simulink model "AdaptiveModel"  (R2017b)
settings: Solver=VariableStepAuto  StartTime=0.0  StopTime=50  RelTol=1e-3
values from neighbouring files (symbols this model uses):
  beta = 40    [init.m]
  d = 1    [PP_rt.m]    (also in Poleplace.m; init.m)
  DT = 25    [init.m]
  Hr = [1 1]    [codegen.m]    (also in init.m)
  Hs = [1 -1]    [codegen.m]    (also in init.m)
  lambda = 0.95    [init.m]
  nA = length(A) - 1    [PP_rt_mauro.m]    (also in init.m)
  nB = length(B)    [PP_rt_mauro.m]    (also in init.m = length(B)-d-1)
  P = conv(P, Pf)    [PP_rt.m]    (also in PP_rt_mauro.m; codegen.m = [1 p1 p2]; init.m = [1 p1 p2])
  R1 = [33.5196767708 -58.8280554104 -1.87387669035 47.8358795149 0.399729759777 -15.7091995028 -25.6032753946 14.884365398 6.95997961448 3.86481013031 -6.742321562 4.41607857048 ... (17 elements, 1x17)]    [K1.mat]    (also in PP_rt.m = x(n_s1+2:end)'; Poleplace.m = x(n_s1+2:end)')
  R2 = [3.1342268844 -8.1399581872 5.33533955505 7.22995752468 -11.9866953907 -6.12499171015 23.0985636543 -12.1704635393 -4.51612658948 4.32936024322 -1.34202391707 6.4773700521 ... (17 elements, 1x17)]    [K2.mat]    (also in codegen.m = R_final)
  R3 = [3.98644760074 -10.644578896 12.4117237154 -5.12999859704 -6.58572397563 12.528754402 -9.78958840161 3.26868202994]    [K3.mat]    (also in K3_with_four_poles.mat = [1.61350975718 -4.21138815342 4.85167932198 -1.93039613093 -; init.m = [R3,0])
  S1 = [1 0.47525789568 -0.120791737843 -0.659025383432 -0.740602287059 -0.383041723471 0.0476399963873 0.338468948565 0.342443506099 0.181293316692 -0.0249270399759 -0.1387227703 ... (16 elements, 1x16)]    [K1.mat]    (also in PP_rt.m = x(1:n_s1+1)'; Poleplace.m = x(1:n_s1+1)')
  S2 = [1 -1.30861512012 -0.251094188933 0.310166607487 0.641482122367 -0.0760817308484 -0.446961768632 0.0650663960157 0.174068991686 -0.0320715572699 -0.0977287236514 -0.0172838591405 ... (16 elements, 1x16)]    [K2.mat]    (also in codegen.m = S_final)
  S3 = [1 -1.72076165185 1.25933960301 -0.482682162577 0.0902319524628 -0.117297255986 -0.0288304850576]    [K3.mat]    (also in K3_with_four_poles.mat = [1 -2.32113674008 2.28108582065 -1.19868534637 0.34993218961; init.m = [S3,0])
  Ts = 0.04    [codegen.m]    (also in init.m; p1p2.m)
libraries: cstblocks x3, simulink x1
settings Model: Creator=akarimi  LastModifiedBy=stenelling
settings CodeAppCC: StateflowObjectComments=on

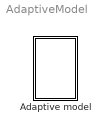
== system AdaptiveModel ==
  Adaptive model : Subsystem

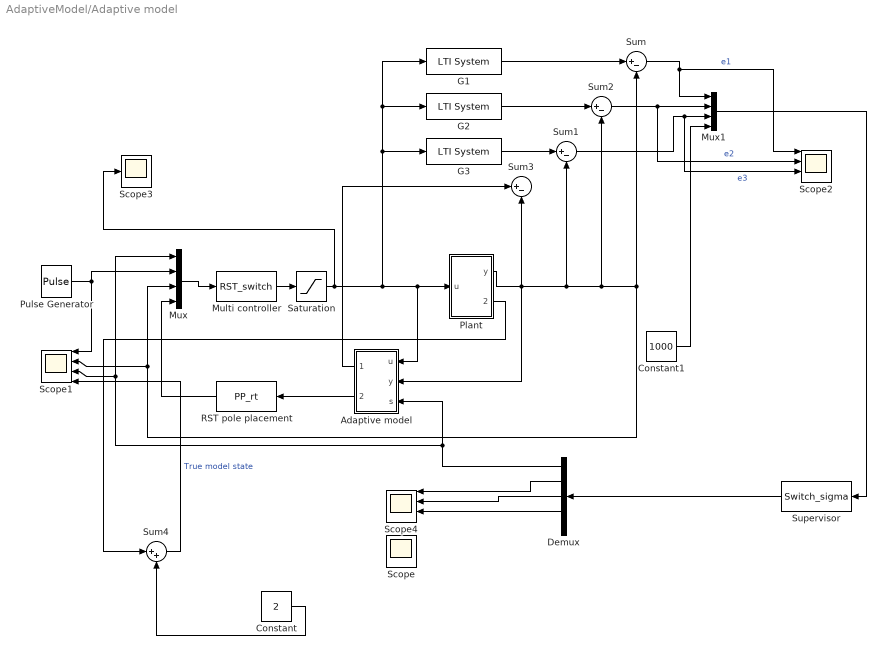
== system AdaptiveModel/Adaptive model ==
  Adaptive model : Subsystem
  Constant : Constant  Value=2
  Constant1 : Constant  Value=1000
  Demux : Demux  Outputs=5
  G1 : cstblocks/LTI System  sys=G1  IC=[]
  G2 : cstblocks/LTI System  sys=G2  IC=[]
  G3 : cstblocks/LTI System  sys=G3  IC=[]
  Multi controller : S-Function  FunctionName=RST_switch  Parameters=R1,S1,R2,S2,R3,S3,Ts  SFunctionDeploymentMode=off  EnableBusSupport=off
  Mux : Mux
  Mux1 : Mux
  Plant : Subsystem
  Pulse Generator : DiscretePulseGenerator  PulseType=Time based  Period=10  PulseWidth=50  PhaseDelay=5
  RST pole placement : S-Function  FunctionName=PP_rt  Parameters=nA,nB,d,P,Hs,Hr,Ts  SFunctionModules='Poleplace'  SFunctionDeploymentMode=off  EnableBusSupport=off
  Saturation : Saturate  UpperLimit=2  LowerLimit=-2
  Scope : Scope
  Scope1 : Scope  NumInputPorts=4
  Scope2 : Scope  NumInputPorts=4
  Scope3 : Scope
  Scope4 : Scope  NumInputPorts=4
  Sum{,1..3} (4 alike) : Sum  Inputs=|+-
  Sum4 : Sum  Inputs=|++
  Supervisor : S-Function  FunctionName=Switch_sigma  Parameters=beta,lambda,DT  SFunctionDeploymentMode=off  EnableBusSupport=off
  wires:
  Mux/1 -> Multi controller/1
  RST pole placement/1 -> Mux/4
  Pulse Generator/1 -> Scope1/1, Mux/2
  Plant/1(y) -> Adaptive model/2(y), Sum3/2, Scope1/2, Mux/3, Sum/2, Sum2/2, Sum1/2
  Multi controller/1 -> Saturation/1
  Adaptive model/2(theta) -> RST pole placement/1
  Adaptive model/1(yhat) -> Sum3/1
  Sum2/1 -> Scope2/2, Mux1/2  "e2"
  Sum/1 -> Scope2/1, Mux1/1  "e1"
  Sum1/1 -> Scope2/3, Mux1/3  "e3"
  Mux1/1 -> Supervisor/1
  G1/1 -> Sum/1
  G2/1 -> Sum2/1
  G3/1 -> Sum1/1
  Demux/1 -> Adaptive model/3(s), Scope1/3, Mux/1
  Plant/2(True) -> Sum4/1
  Constant/1 -> Sum4/2
  Sum4/1 -> Scope1/4  "True model state"
  Saturation/1 -> Scope3/1, G1/1, G2/1, G3/1, Adaptive model/1(u), Plant/1(u)
  Constant1/1 -> Mux1/4
  Supervisor/1 -> Demux/1
  Demux/2 -> Scope4/1
  Demux/3 -> Scope4/2
  Demux/4 -> Scope4/3

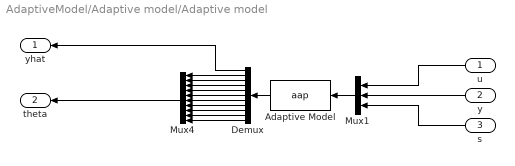
== system AdaptiveModel/Adaptive model/Adaptive model ==
  u : Inport
  y : Inport  Port=2
  s : Inport  Port=3
  "Adaptive Model " : S-Function  FunctionName=aap  Parameters=nA,nB,d  SFunctionDeploymentMode=off  EnableBusSupport=off
  Demux : Demux  Outputs=11
  Mux1 : Mux  Inputs=3
  Mux4 : Mux  Inputs=10
  yhat : Outport
  theta : Outport  Port=2
  wires:
  Mux1/1 -> "Adaptive Model "/1
  Mux4/1 -> theta/1
  Demux/3 -> Mux4/2
  Demux/9 -> Mux4/8
  Demux/8 -> Mux4/7
  y/1 -> Mux1/2
  Demux/4 -> Mux4/3
  Demux/5 -> Mux4/4
  "Adaptive Model "/1 -> Demux/1
  Demux/10 -> Mux4/9
  u/1 -> Mux1/1
  Demux/1 -> yhat/1
  Demux/2 -> Mux4/1
  Demux/7 -> Mux4/6
  Demux/11 -> Mux4/10
  Demux/6 -> Mux4/5
  s/1 -> Mux1/3

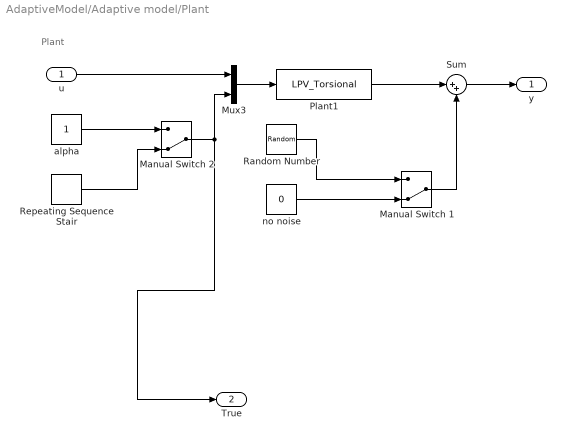
== system AdaptiveModel/Adaptive model/Plant ==
  note: Plant
  u : Inport
  Manual Switch 1 : ManualSwitch  CurrentSetting=0
  Manual Switch 2 : ManualSwitch  CurrentSetting=0
  Mux3 : Mux  Inputs=2
  Plant1 : S-Function  FunctionName=LPV_Torsional  SFunctionDeploymentMode=off  EnableBusSupport=off
  Random Number : RandomNumber  Variance=0.00001  SampleTime=Ts
  Repeating Sequence Stair : simulink/Sources/Repeating Sequence Stair  OutValues="[ -1 1  ].'"  tsamp=25  OutMin=[]  OutMax=[]  OutDataTypeStr=double  OutputDataTypeScalingMode=double  OutDataType=fixdt(0,8)  ConRadixGroup=Best Precision: Vector-wise  OutScaling=2^-12
  Sum : Sum  Inputs=|++
  alpha : Constant
  "no noise " : Constant  Value=0
  y : Outport
  True : Outport  Port=2
  wires:
  Sum/1 -> y/1
  Random Number/1 -> Manual Switch 1/1
  u/1 -> Mux3/1
  Repeating Sequence Stair/1 -> Manual Switch 2/2
  Mux3/1 -> Plant1/1
  Plant1/1 -> Sum/1
  Manual Switch 1/1 -> Sum/2
  Manual Switch 2/1 -> Mux3/2, True/1
  "no noise "/1 -> Manual Switch 1/2
  alpha/1 -> Manual Switch 2/1
